simulink library "mr_thrust"  (R2022b)
settings: Solver=VariableStepAuto  StartTime=0.0  StopTime=10.0  RelTol=1e-3
undefined symbols (not defined in the file or in its folder): plant_sample_time_s, veh_params
settings Model: Creator=Tanmay.Mandal  LastModifiedBy=Tanmay.Mandal

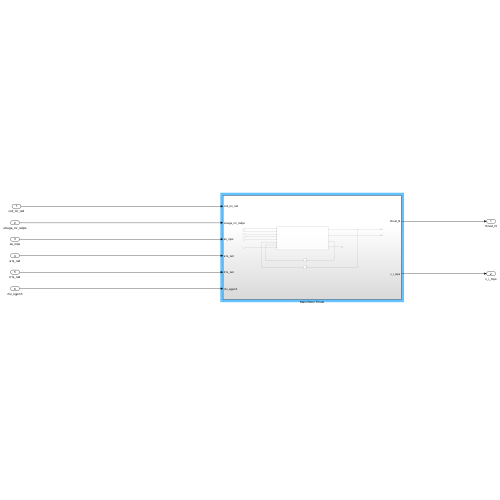
[thumbnail: Simulink's stored preview of the top-level diagram]
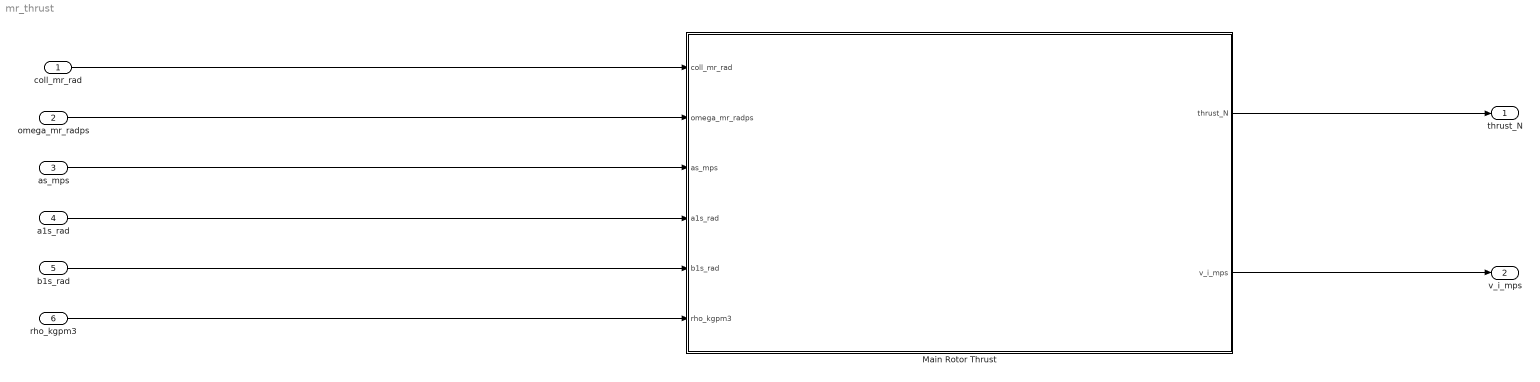
== system mr_thrust ==
  coll_mr_rad : Inport  OutDataTypeStr=double  Unit=rad  PortDimensions=1
  omega_mr_radps : Inport  Port=2  OutDataTypeStr=double  Unit=rad/s  PortDimensions=1
  as_mps : Inport  Port=3  OutDataTypeStr=double  Unit=m/s  PortDimensions=[3, 1]
  a1s_rad : Inport  Port=4  OutDataTypeStr=double  Unit=rad  PortDimensions=1
  b1s_rad : Inport  Port=5  OutDataTypeStr=double  Unit=rad  PortDimensions=1
  rho_kgpm3 : Inport  Port=6  OutDataTypeStr=double  Unit=kg/m^3  PortDimensions=1
  Main Rotor Thrust : Subsystem
  thrust_N : Outport  OutDataTypeStr=double  Unit=1  PortDimensions=N
  v_i_mps : Outport  Port=2  OutDataTypeStr=double  Unit=m/s  PortDimensions=1
  wires:
  coll_mr_rad/1 -> Main Rotor Thrust/1(coll_mr_rad)
  omega_mr_radps/1 -> Main Rotor Thrust/2(omega_mr_radps)
  as_mps/1 -> Main Rotor Thrust/3(as_mps)
  a1s_rad/1 -> Main Rotor Thrust/4(a1s_rad)
  b1s_rad/1 -> Main Rotor Thrust/5(b1s_rad)
  rho_kgpm3/1 -> Main Rotor Thrust/6(rho_kgpm3)
  Main Rotor Thrust/1(thrust_N) -> thrust_N/1
  Main Rotor Thrust/2(v_i_mps) -> v_i_mps/1

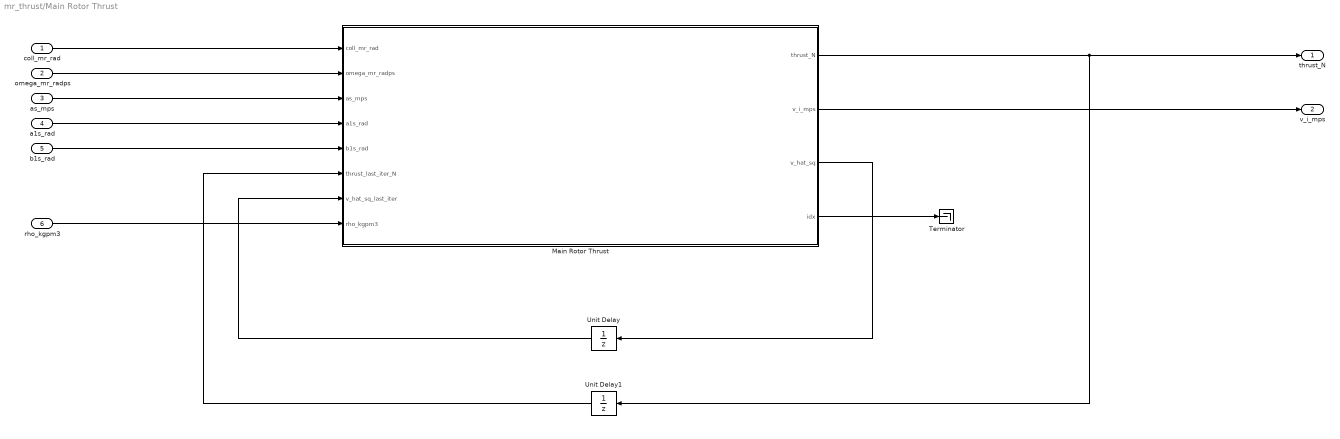
== system mr_thrust/Main Rotor Thrust ==
  coll_mr_rad : Inport
  omega_mr_radps : Inport  Port=2
  as_mps : Inport  Port=3
  a1s_rad : Inport  Port=4
  b1s_rad : Inport  Port=5
  rho_kgpm3 : Inport  Port=6
  Main Rotor Thrust : MATLAB Function  TreatAsAtomicUnit=on  mask{params=veh_params.main_rotor}
      mask prompts: params "Main Rotor Params Struct"
  Terminator : Terminator
  Unit Delay : UnitDelay  InitialCondition=-1  SampleTime=plant_sample_time_s  HasFrameUpgradeWarning=on
  Unit Delay1 : UnitDelay  InitialCondition=-1  SampleTime=plant_sample_time_s  HasFrameUpgradeWarning=on
  thrust_N : Outport
  v_i_mps : Outport  Port=2  OutDataTypeStr=double  Unit=m/s  PortDimensions=1
  wires:
  b1s_rad/1 -> Main Rotor Thrust/5(b1s_rad)
  Unit Delay1/1 -> Main Rotor Thrust/6(thrust_last_iter_N)
  Main Rotor Thrust/1(thrust_N) -> Unit Delay1/1, thrust_N/1
  as_mps/1 -> Main Rotor Thrust/3(as_mps)
  rho_kgpm3/1 -> Main Rotor Thrust/8(rho_kgpm3)
  Main Rotor Thrust/4(idx) -> Terminator/1
  Unit Delay/1 -> Main Rotor Thrust/7(v_hat_sq_last_iter)
  Main Rotor Thrust/3(v_hat_sq) -> Unit Delay/1
  coll_mr_rad/1 -> Main Rotor Thrust/1(coll_mr_rad)
  a1s_rad/1 -> Main Rotor Thrust/4(a1s_rad)
  omega_mr_radps/1 -> Main Rotor Thrust/2(omega_mr_radps)
  Main Rotor Thrust/2(v_i_mps) -> v_i_mps/1

== matlab function mr_thrust/Main Rotor Thrust/Main Rotor Thrust ==
  data: coll_mr_rad input double size=1; thrust_N output double size=1; v_i_mps output double; omega_mr_radps input double size=1; as_mps input size=[3, 1]; a1s_rad input double size=1; b1s_rad input double size=1; thrust_last_iter_N input size=1; v_hat_sq_last_iter input double size=1; rho_kgpm3 input size=1; v_hat_sq output double size=1; idx output size=1; params parameter
function [thrust_N, v_i_mps, v_hat_sq, idx] = thrust_dynamics(coll_mr_rad, omega_mr_radps, as_mps, ...
                            a1s_rad, b1s_rad, thrust_last_iter_N, v_hat_sq_last_iter, rho_kgpm3, params)
%THRUST_DYNAMICS_FUNCTION Computes main rotor thrust based on classical
%momentum theory
%
%Inputs:
%coll_mr_rad                    : Collective command
%omega_mr_radps                 : Main rotor angular velocity
%as_mps                         : Airspeed vector in body axis
%a1s_rad                        : Longitudinal flap angle
%b1s_rad                        : Lateral flap angle
%thrust_last_iter_N             : Computed thrust from last simulation
%                                 iteration
%v_hat_sq_last_iter             : Computed v_hat_sq from last simulation
%                                 iteration
%rho_kgpm3                      : Altitude corrected air density
%params                         : Main rotor parameters struct
%
%Outputs:
%thrust_N                       : Computed main rotor thrust
%v_i_mps                        : Induced velocity at main rotor
%v_hat_sq                       : Computed v_hat_sq
%idx                            : Iteration index when solution converged
%                                 for debug purpose

[thrust_N, v_i_mps, v_hat_sq, idx] = thrust_dynamics_function(coll_mr_rad, omega_mr_radps, as_mps, ...
                            a1s_rad, b1s_rad, thrust_last_iter_N, v_hat_sq_last_iter, rho_kgpm3, params);
